simulink model "Potoo_Dyn_Model_v3px4_Flap_compact"  (R2024b)
settings: Solver=FixedStepAuto  StartTime=0.0  StopTime=120  FixedStep=0.001  MaxStep=0.001  RelTol=1e-3
InitFcn:
  | Tmech = 0.004;
undefined symbols (not defined in the file): Control, custom_ff, DiscIntNeverNeededParam, Earth, F, fractalcoef, Light, MIL, Potoo, Px4_Parms, realflap, tau, theta_max, thetadot_max, WGS84
libraries: cstblocks x10, matrix_library x10, aerolibasang x7, simulink x6, aerolibadyn x3, sharedtransform x2, slctrl_autotuning x1, mspfiltlib x1, mspsensorlib x1, shared6dof x1, aerolibactuator x1, aerolibatmos2 x1
(part 2 of 2)

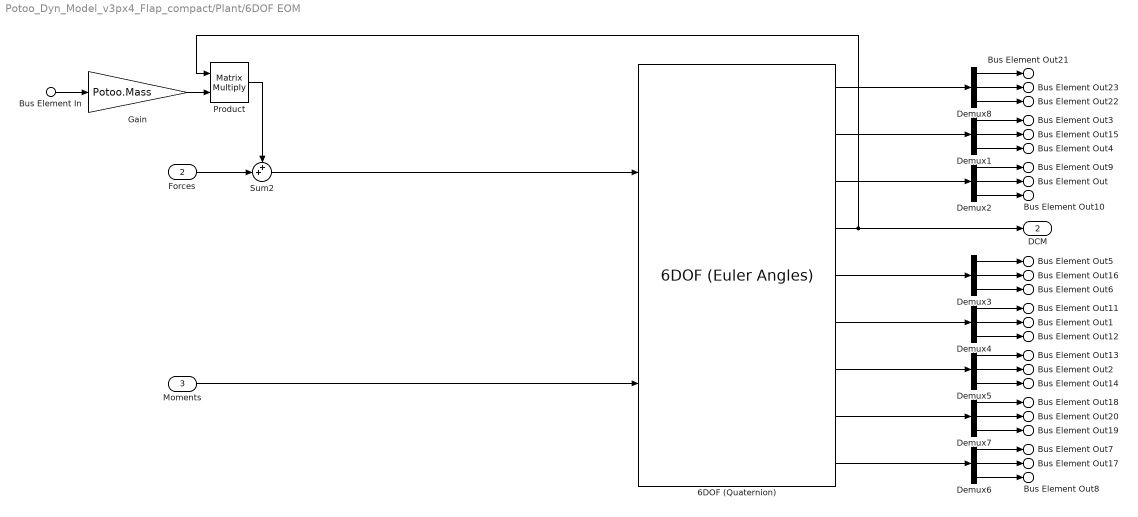
== system Potoo_Dyn_Model_v3px4_Flap_compact/Plant/6DOF EOM ==
  Bus Element In : Inport  PortName=Env  Element=g
  Forces : Inport  Port=2
  Moments : Inport  Port=3
  6DOF (Quaternion) : shared6dof/6DOF (Euler Angles)  units=English (Velocity in ft/s)  mtype=Fixed  rep=Quaternion  xme_0=IC.P_0  Vm_0=IC.V_0  eul_0=IC.E_0  pm_0=IC.omega_0  mass_0=Potoo.Mass  mass_e=0.5  mass_f=2.0  inertia=Potoo.Inertia  inertia_e=eye(3)  inertia_f=2*eye(3)  k_quat=1.0  vre_flag=on  abi_flag=on  aMode=0  xme_statename=''  Vm_statename=''  eul_statename=''  quat_statename=''  pm_statename=''  mass_statename=''
      settings: LibrarySourceBlock=aerolib6dof2/6DOF (Quaternion)
  Demux{1..8} (8 alike) : Demux  Outputs=3
  Gain : Gain  Gain=Potoo.Mass
  Product : Product  Multiplication=Matrix(*)
  Sum2 : Sum  Inputs=++|  InputSameDT=on  SaturateOnIntegerOverflow=on  OutDataTypeStr=Inherit: Same as first input
  Bus Element Out3 : Outport  VectorParamsAs1DForOutWhenUnconnected=off  PortName=States  Element=Xe
  Bus Element Out4 : Outport  VectorParamsAs1DForOutWhenUnconnected=off  PortName=States  Element=Ze
  Bus Element Out : Outport  VectorParamsAs1DForOutWhenUnconnected=off  PortName=States  Element=theta
  Bus Element Out5 : Outport  VectorParamsAs1DForOutWhenUnconnected=off  PortName=States  Element=u
  Bus Element Out6 : Outport  VectorParamsAs1DForOutWhenUnconnected=off  PortName=States  Element=w
  Bus Element Out1 : Outport  VectorParamsAs1DForOutWhenUnconnected=off  PortName=States  Element=q
  Bus Element Out2 : Outport  VectorParamsAs1DForOutWhenUnconnected=off  PortName=States  Element=q_dot
  Bus Element Out7 : Outport  VectorParamsAs1DForOutWhenUnconnected=off  PortName=States  Element=Axe
  Bus Element Out8 : Outport  VectorParamsAs1DForOutWhenUnconnected=off  PortName=States  Element=Aze
  Bus Element Out15 : Outport  VectorParamsAs1DForOutWhenUnconnected=off  PortName=States  Element=Ye
  Bus Element Out9 : Outport  VectorParamsAs1DForOutWhenUnconnected=off  PortName=States  Element=phi
  Bus Element Out10 : Outport  VectorParamsAs1DForOutWhenUnconnected=off  PortName=States  Element=psi
  Bus Element Out16 : Outport  VectorParamsAs1DForOutWhenUnconnected=off  PortName=States  Element=v
  Bus Element Out11 : Outport  VectorParamsAs1DForOutWhenUnconnected=off  PortName=States  Element=p
  Bus Element Out12 : Outport  VectorParamsAs1DForOutWhenUnconnected=off  PortName=States  Element=r
  Bus Element Out13 : Outport  VectorParamsAs1DForOutWhenUnconnected=off  PortName=States  Element=p_dot
  Bus Element Out14 : Outport  VectorParamsAs1DForOutWhenUnconnected=off  PortName=States  Element=r_dot
  Bus Element Out17 : Outport  VectorParamsAs1DForOutWhenUnconnected=off  PortName=States  Element=Aye
  Bus Element Out18 : Outport  VectorParamsAs1DForOutWhenUnconnected=off  PortName=States  Element=u_dot
  Bus Element Out19 : Outport  VectorParamsAs1DForOutWhenUnconnected=off  PortName=States  Element=w_dot
  Bus Element Out20 : Outport  VectorParamsAs1DForOutWhenUnconnected=off  PortName=States  Element=v_dot
  Bus Element Out21 : Outport  VectorParamsAs1DForOutWhenUnconnected=off  PortName=States  Element=Vxe
  Bus Element Out22 : Outport  VectorParamsAs1DForOutWhenUnconnected=off  PortName=States  Element=Vze
  Bus Element Out23 : Outport  VectorParamsAs1DForOutWhenUnconnected=off  PortName=States  Element=Vye
  DCM : Outport  Port=2
  wires:
  Demux6/2 -> Bus Element Out17/1
  Demux6/3 -> Bus Element Out8/1
  Demux6/1 -> Bus Element Out7/1
  Demux5/3 -> Bus Element Out14/1
  Demux5/2 -> Bus Element Out2/1
  Demux5/1 -> Bus Element Out13/1
  Demux4/3 -> Bus Element Out12/1
  Demux4/2 -> Bus Element Out1/1
  Demux4/1 -> Bus Element Out11/1
  Demux3/3 -> Bus Element Out6/1
  Demux3/2 -> Bus Element Out16/1
  Demux3/1 -> Bus Element Out5/1
  Demux2/3 -> Bus Element Out10/1
  Demux2/2 -> Bus Element Out/1
  Demux2/1 -> Bus Element Out9/1
  Demux1/1 -> Bus Element Out3/1
  Demux1/3 -> Bus Element Out4/1
  Demux1/2 -> Bus Element Out15/1
  Forces/1 -> Sum2/2
  Product/1 -> Sum2/1
  6DOF (Quaternion)/8 -> Demux7/1
  6DOF (Quaternion)/9 -> Demux6/1
  6DOF (Quaternion)/2 -> Demux1/1
  6DOF (Quaternion)/3 -> Demux2/1
  6DOF (Quaternion)/7 -> Demux5/1
  6DOF (Quaternion)/6 -> Demux4/1
  6DOF (Quaternion)/5 -> Demux3/1
  Sum2/1 -> 6DOF (Quaternion)/1
  Moments/1 -> 6DOF (Quaternion)/2
  Demux7/3 -> Bus Element Out19/1
  Demux7/2 -> Bus Element Out20/1
  Demux7/1 -> Bus Element Out18/1
  Demux8/1 -> Bus Element Out21/1
  Demux8/3 -> Bus Element Out22/1
  Demux8/2 -> Bus Element Out23/1
  6DOF (Quaternion)/1 -> Demux8/1
  Bus Element In/1 -> Gain/1
  6DOF (Quaternion)/4 -> DCM/1, Product/1
  Gain/1 -> Product/2

== system Potoo_Dyn_Model_v3px4_Flap_compact/Plant/Aerodynamic Model ==
  Env : Inport
  ActuatorCmds : Inport  Port=2  OutDataTypeStr=Bus: ActuatorCmds  PortDimensions=4
  States : Inport  Port=3
  Add : Sum  Inputs=+++++
  Add1 : Sum  Inputs=+++++
  Demux : Demux
  Demux1 : Demux
  For Each Subsystem : Subsystem  TreatAsAtomicUnit=on  mask{wingStruct=[Potoo.Wings.Wing1,Potoo.Wings.Wing2,Potoo.Wings.Wing3,Potoo.Wings.Wing4]}
      mask prompts: wingStruct "Wing Structure"
  Fueslage : Subsystem
  F : Outport  Unit=lbf  VectorParamsAs1DForOutWhenUnconnected=off
  M : Outport  Port=2  Unit=ft*lbf  VectorParamsAs1DForOutWhenUnconnected=off
  wires:
  Add/1 -> F/1
  Add1/1 -> M/1
  States/1 -> For Each Subsystem/3(States)
  ActuatorCmds/1 -> For Each Subsystem/2(Actuator Comands)
  Env/1 -> For Each Subsystem/1(Env)
  For Each Subsystem/1(F) -> Demux/1
  For Each Subsystem/2(M) -> Demux1/1
  Demux/1 -> Add/2
  Demux/2 -> Add/3
  Demux/3 -> Add/4
  Demux/4 -> Add/5
  Demux1/1 -> Add1/1
  Demux1/2 -> Add1/2
  Demux1/3 -> Add1/3
  Demux1/4 -> Add1/4

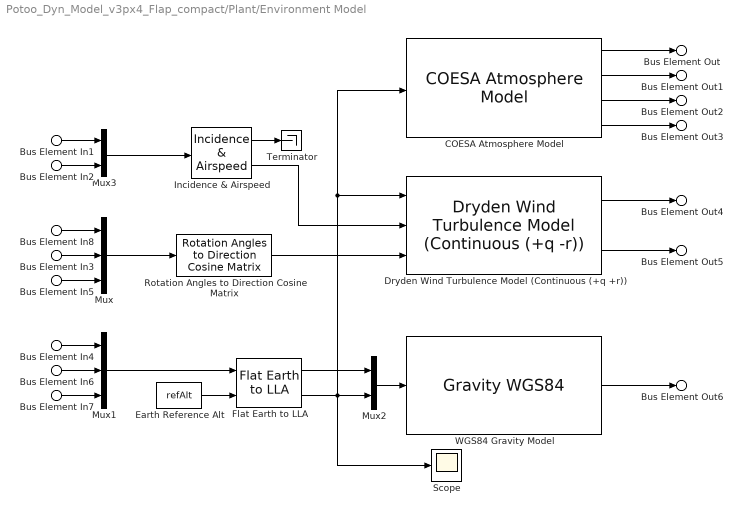
== system Potoo_Dyn_Model_v3px4_Flap_compact/Plant/Environment Model ==
  Bus Element In1 : Inport  PortName=States  Element=u
  Bus Element In2 : Inport  PortName=States  Element=w
  Bus Element In3 : Inport  PortName=States  Element=theta
  Bus Element In4 : Inport  PortName=States  Element=Xe
  Bus Element In7 : Inport  PortName=States  Element=Ze
  Bus Element In8 : Inport  PortName=States  Element=phi
  Bus Element In5 : Inport  PortName=States  Element=psi
  Bus Element In6 : Inport  PortName=States  Element=Ye
  COESA Atmosphere Model : aerolibatmos2/COESA Atmosphere Model  units=English (Velocity in ft/s)  spec=1976 COESA-extended U.S. Standard Atmosphere  model=Profile  profile_var=High temperature  profile_percent=1%  profile_alt=5 km (16404 ft)  envelope_var=High temperature  envelope_percent=1%  action=Warning
  Dryden Wind Turbulence Model (Continuous (+q +r)) : aerolibwind2/Dryden Wind Turbulence Model  (Continuous (+q -r))  units=English (Velocity in ft/s)  spec=MIL-F-8785C  model=Continuous Dryden (+q -r)  W20=W20  Wdeg=Wdeg  TurbProb=10^-2 - Light  L_high=L_high  Wingspan=Wingspan  ts=ts  Seed=Seed  T_on=off
  Earth Reference Alt : Constant  Value=refAlt
  Flat Earth to LLA : aerolibtransform2/Flat Earth to LLA  units=English  ptype=Earth (WGS84)  F=1/298.257223563  R=20925646.3255  refPosPort=off  LL0=[0 0]  psi=0
  Incidence & Airspeed : aerolibasang/Incidence  & Airspeed
  Mux : Mux  Inputs=3
  Mux1 : Mux  Inputs=3
  Mux2 : Mux  Inputs=2
  Mux3 : Mux  Inputs=2
  Rotation Angles to Direction Cosine Matrix : sharedtransform/Rotation Angles to Direction Cosine Matrix  rotationOrder=ZYX  aMode=aMode
  Scope : Scope
  Terminator : Terminator
  "WGS84 Gravity Model  " : GravityWGS84  units=English
  Bus Element Out : Outport  VectorParamsAs1DForOutWhenUnconnected=off  PortName=Env  Element=To
  Bus Element Out1 : Outport  VectorParamsAs1DForOutWhenUnconnected=off  PortName=Env  Element=a
  Bus Element Out2 : Outport  VectorParamsAs1DForOutWhenUnconnected=off  PortName=Env  Element=Po
  Bus Element Out3 : Outport  VectorParamsAs1DForOutWhenUnconnected=off  PortName=Env  Element=AirDensity
  Bus Element Out4 : Outport  VectorParamsAs1DForOutWhenUnconnected=off  PortName=Env  Element=WindVelocity
  Bus Element Out5 : Outport  VectorParamsAs1DForOutWhenUnconnected=off  PortName=Env  Element=WindAngularRates
  Bus Element Out6 : Outport  VectorParamsAs1DForOutWhenUnconnected=off  PortName=Env  Element=g
  wires:
  Dryden Wind Turbulence Model (Continuous (+q +r))/1 -> Bus Element Out4/1
  Dryden Wind Turbulence Model (Continuous (+q +r))/2 -> Bus Element Out5/1
  Mux2/1 -> "WGS84 Gravity Model  "/1
  Bus Element In4/1 -> Mux1/1
  Bus Element In7/1 -> Mux1/3
  Bus Element In6/1 -> Mux1/2
  Bus Element In5/1 -> Mux/3
  Bus Element In8/1 -> Mux/1
  Bus Element In2/1 -> Mux3/2
  Bus Element In1/1 -> Mux3/1
  "WGS84 Gravity Model  "/1 -> Bus Element Out6/1
  COESA Atmosphere Model/2 -> Bus Element Out1/1
  COESA Atmosphere Model/1 -> Bus Element Out/1
  COESA Atmosphere Model/4 -> Bus Element Out3/1
  COESA Atmosphere Model/3 -> Bus Element Out2/1
  Flat Earth to LLA/1 -> Mux2/1
  Earth Reference Alt/1 -> Flat Earth to LLA/2
  Incidence & Airspeed/2 -> Dryden Wind Turbulence Model (Continuous (+q +r))/2
  Flat Earth to LLA/2 -> Scope/1, Mux2/2, COESA Atmosphere Model/1, Dryden Wind Turbulence Model (Continuous (+q +r))/1
  Mux3/1 -> Incidence & Airspeed/1
  Incidence & Airspeed/1 -> Terminator/1
  Mux/1 -> Rotation Angles to Direction Cosine Matrix/1
  Bus Element In3/1 -> Mux/2
  Rotation Angles to Direction Cosine Matrix/1 -> Dryden Wind Turbulence Model (Continuous (+q +r))/3
  Mux1/1 -> Flat Earth to LLA/1

== system Potoo_Dyn_Model_v3px4_Flap_compact/Controller/Attitude Controller/Norm3 ==
  In1 : Inport
  Dot Product : DotProduct  OutDataTypeStr=Inherit: Inherit via internal rule
  Math Function1 : Math  Operator=sqrt  SignedPower=on
  Out1 : Outport  VectorParamsAs1DForOutWhenUnconnected=off
  wires:
  Dot Product/1 -> Math Function1/1
  Math Function1/1 -> Out1/1
  In1/1 -> Dot Product/1, Dot Product/2

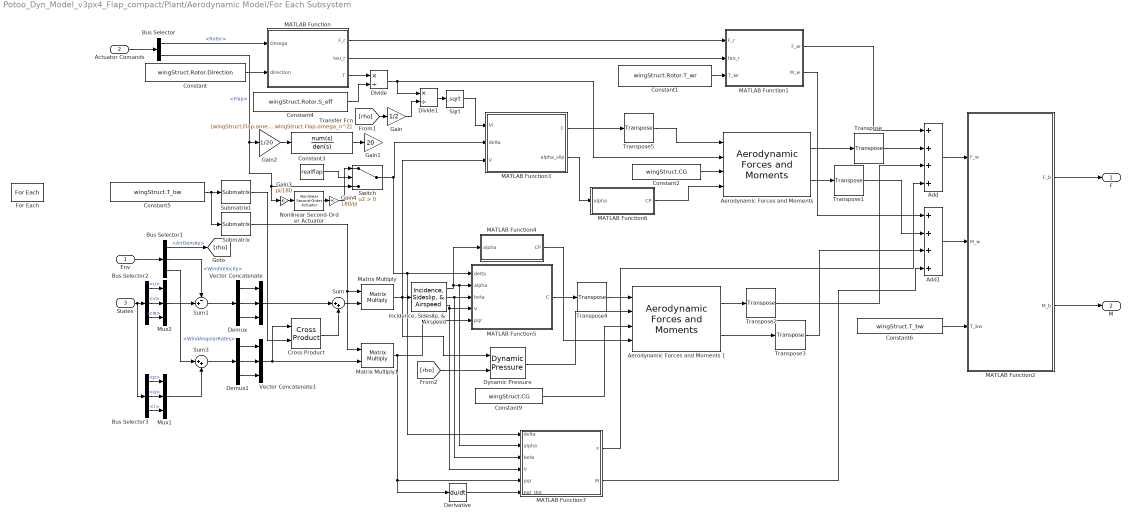
== system Potoo_Dyn_Model_v3px4_Flap_compact/Plant/Aerodynamic Model/For Each Subsystem ==
  Env : Inport
  Actuator Comands : Inport  Port=2  Partition=on  PartitionDimension=1  PartitionWidth=1  PartitionOffset=0
  States : Inport  Port=3
  Add : Sum  Inputs=++++
  Add1 : Sum  Inputs=++++
  "Aerodynamic Forces and Moments " : aerolibadyn/Aerodynamic Forces and Moments   inputAxes=Body  outputForceAxes=Body  outputMomentAxes=Body  S=wingStruct.Rotor.S_eff  b=Potoo.ReferenceSpan  cbar=Potoo.ReferenceLength
  Aerodynamic Forces and Moments 1 : aerolibadyn/Aerodynamic Forces and Moments   inputAxes=Body  outputForceAxes=Body  outputMomentAxes=Body  S=Potoo.ReferenceArea  b=Potoo.ReferenceSpan  cbar=Potoo.ReferenceLength
  Bus Selector : BusSelector  OutputSignals=Rotor,Flap
  Bus Selector1 : BusSelector  OutputSignals=AirDensity,WindVelocity,WindAngularRates
  Bus Selector2 : BusSelector  OutputSignals=u,v,w
  Bus Selector3 : BusSelector  OutputSignals=p,q,r
  Constant : Constant  Value=wingStruct.Rotor.Direction
  Constant1 : Constant  Value=wingStruct.Rotor.T_wr
  Constant2 : Constant  Value=wingStruct.CG
  Constant3 : Constant  Value=realflap
  Constant4 : Constant  Value=wingStruct.Rotor.S_eff
  Constant5 : Constant  Value=wingStruct.T_bw
  Constant6 : Constant  Value=wingStruct.T_bw
  Constant9 : Constant  Value=wingStruct.CG
  Cross Product : matrix_library/Cross Product
  Demux : Demux  Outputs=3
  Demux1 : Demux  Outputs=3
  Derivative : Derivative
  Divide : Product  Inputs=*/
  Divide1 : Product  Inputs=*/
  Dynamic Pressure : aerolibasang/Dynamic Pressure
  For Each : ForEach  DisableCoverage=on  IterateSubsysMaskParameter=on  SubsysMaskParameterIterationDimension=2
  Gain : Gain  Gain=1/2
  Gain1 : Gain  Gain=20
  Gain2 : Gain  Gain=1/20
  Gain3 : Gain  Gain=pi/180
  Gain4 : Gain  Gain=180/pi
  "Incidence, Sideslip, & Airspeed" : aerolibasang/Incidence, Sideslip, & Airspeed
  MATLAB Function : MATLAB Function  TreatAsAtomicUnit=on
  MATLAB Function1 : MATLAB Function  TreatAsAtomicUnit=on
  MATLAB Function2 : MATLAB Function  TreatAsAtomicUnit=on
  MATLAB Function3 : MATLAB Function  TreatAsAtomicUnit=on
  MATLAB Function4 : MATLAB Function  TreatAsAtomicUnit=on
  MATLAB Function5 : MATLAB Function  TreatAsAtomicUnit=on
  MATLAB Function6 : MATLAB Function  TreatAsAtomicUnit=on
  MATLAB Function7 : MATLAB Function  TreatAsAtomicUnit=on
  Matrix Multiply : Product  Multiplication=Matrix(*)
  Matrix Multiply1 : Product  Multiplication=Matrix(*)
  Mux1 : Mux  Inputs=3
  Mux2 : Mux  Inputs=3
  Nonlinear Second-Order Actuator : aerolibactuator/Nonlinear Second-Order Actuator  wn_fin=omega_n  z_fin=zeta  fin_max=theta_max*pi/180  fin_min=-theta_max*pi/180  fin_maxrate=thetadot_max*pi/180  fin_act_0=0  fin_act_vel=0
  Sqrt : Sqrt
  Submatrix : matrix_library/Submatrix  RowSpan=Range of rows  RowStartMode=First  RowStartIndex=1  RowEndMode=Offset from last  RowEndIndex=1  ColSpan=Range of columns  ColStartMode=First  ColStartIndex=1  ColEndMode=Offset from last  ColEndIndex=1
  Submatrix1 : matrix_library/Submatrix  RowSpan=Range of rows  RowStartMode=First  RowStartIndex=1  RowEndMode=Offset from last  RowEndIndex=1  ColSpan=Range of columns  ColStartMode=Last  ColStartIndex=1  ColEndMode=Offset from last  ColEndIndex=1
  Sum : Sum  Inputs=|++
  Sum1 : Sum  Inputs=-+|  InputSameDT=on  SaturateOnIntegerOverflow=on  OutDataTypeStr=Inherit: Same as first input
  Sum3 : Sum  Inputs=|++  InputSameDT=on  SaturateOnIntegerOverflow=on  OutDataTypeStr=Inherit: Same as first input
  Switch : Switch  Criteria=u2 > Threshold  SaturateOnIntegerOverflow=off  InputSameDT=off
  Transfer Fcn : TransferFcn  Numerator=[wingStruct.Flap.omega_n^2]  Denominator=[1 2*wingStruct.Flap.omega_n wingStruct.Flap.omega_n^2]
  Transpose{,1..5} (6 alike) : matrix_library/Transpose
  Vector Concatenate : Concatenate  NumInputs=3
  Vector Concatenate1 : Concatenate  NumInputs=3
  F : Outport  Unit=N  ConcatenationDimension=1  VectorParamsAs1DForOutWhenUnconnected=off
  M : Outport  Port=2  Unit=N*m  ConcatenationDimension=1  VectorParamsAs1DForOutWhenUnconnected=off
  wires:
  Bus Selector3/2 -> Mux1/2  "<q>"
  Bus Selector2/2 -> Mux2/2  "<v>"
  Bus Selector3/3 -> Mux1/3  "<r>"
  Bus Selector1/3 -> Sum3/1  "<WindAngularRates>"
  Bus Selector2/1 -> Mux2/1  "<u>"
  Env/1 -> Bus Selector1/1
  [rho] -> Dynamic Pressure/2
  Bus Selector2/3 -> Mux2/3  "<w>"
  States/1 -> Bus Selector3/1, Bus Selector2/1
  Bus Selector1/1 -> [rho]  "<AirDensity>"
  MATLAB Function/2(tau_r) -> MATLAB Function1/2(tau_r)
  MATLAB Function2/2(M_b) -> M/1
  Mux2/1 -> Sum1/2
  Constant2/1 -> "Aerodynamic Forces and Moments "/3
  Demux1/1 -> Vector Concatenate1/1
  Transpose3/1 -> Add1/3
  Constant4/1 -> Divide/2
  Dynamic Pressure/1 -> Aerodynamic Forces and Moments 1/2
  Demux/2 -> Vector Concatenate/2
  "Aerodynamic Forces and Moments "/2 -> Transpose1/1
  Sum3/1 -> Demux1/1
  Demux/3 -> Vector Concatenate/3
  Constant6/1 -> MATLAB Function2/3(T_bw)
  Sum1/1 -> Demux/1
  "Incidence, Sideslip, & Airspeed"/2 -> MATLAB Function5/3(beta), MATLAB Function7/3(beta)
  Add1/1 -> MATLAB Function2/2(M_w)
  Mux1/1 -> Sum3/2
  Demux1/3 -> Vector Concatenate1/3
  MATLAB Function5/1(C) -> Transpose4/1
  MATLAB Function1/2(M_w) -> Add1/1
  Submatrix/1 -> Matrix Multiply/1, Matrix Multiply1/1
  MATLAB Function1/1(F_w) -> Add/1
  Transpose4/1 -> Aerodynamic Forces and Moments 1/1
  MATLAB Function3/1(C) -> Transpose5/1
  Add/1 -> MATLAB Function2/1(F_w)
  Transpose1/1 -> Add1/2
  Constant/1 -> MATLAB Function/2(direction)
  Matrix Multiply1/1 -> MATLAB Function7/5(pqr), Derivative/1, MATLAB Function5/5(pqr)
  Actuator Comands/1 -> Bus Selector/1
  MATLAB Function/3(T) -> Divide/1
  Sum/1 -> Matrix Multiply/2
  Vector Concatenate1/1 -> Matrix Multiply1/2, Cross Product/1
  Demux/1 -> Vector Concatenate/1
  Constant5/1 -> Submatrix/1, Submatrix1/1
  Constant1/1 -> MATLAB Function1/3(T_wr)
  Transpose/1 -> Add/2
  "Incidence, Sideslip, & Airspeed"/3 -> MATLAB Function5/4(V), MATLAB Function7/4(V)
  Divide/1 -> Divide1/1, "Aerodynamic Forces and Moments "/2
  "Aerodynamic Forces and Moments "/1 -> Transpose/1
  Submatrix1/1 -> Cross Product/2
  Matrix Multiply/1 -> MATLAB Function3/3(V), "Incidence, Sideslip, & Airspeed"/1, Dynamic Pressure/1
  Constant9/1 -> Aerodynamic Forces and Moments 1/3
  MATLAB Function2/1(F_b) -> F/1
  Bus Selector3/1 -> Mux1/1  "<p>"
  Cross Product/1 -> Sum/2
  Demux1/2 -> Vector Concatenate1/2
  MATLAB Function4/1(CP) -> Aerodynamic Forces and Moments 1/4
  Vector Concatenate/1 -> Sum/1
  Aerodynamic Forces and Moments 1/1 -> Transpose2/1
  MATLAB Function/1(F_r) -> MATLAB Function1/1(F_r)
  Bus Selector1/2 -> Sum1/1  "<WindVelocity>"
  Aerodynamic Forces and Moments 1/2 -> Transpose3/1
  Bus Selector/1 -> MATLAB Function/1(Omega)  "<Rotor>"
  Transpose2/1 -> Add/3
  Transpose5/1 -> "Aerodynamic Forces and Moments "/1
  [rho] -> Gain/1
  Gain/1 -> Divide1/2
  Divide1/1 -> Sqrt/1
  Sqrt/1 -> MATLAB Function3/1(Vi)
  MATLAB Function6/1(CP) -> "Aerodynamic Forces and Moments "/4
  "Incidence, Sideslip, & Airspeed"/1 -> MATLAB Function5/2(alpha), MATLAB Function7/2(alpha), MATLAB Function4/1(alpha)
  MATLAB Function3/2(alpha_slip) -> MATLAB Function6/1(alpha)
  Bus Selector/2 -> Gain2/1, Switch/3, Gain3/1  "<Flap>"
  MATLAB Function7/1(F) -> Add/4
  MATLAB Function7/2(M) -> Add1/4
  Derivative/1 -> MATLAB Function7/6(pqr_dot)
  Gain2/1 -> Transfer Fcn/1
  Transfer Fcn/1 -> Gain1/1
  Switch/1 -> MATLAB Function7/1(delta), MATLAB Function5/1(delta), MATLAB Function3/2(delta)
  Constant3/1 -> Switch/2
  Gain3/1 -> Nonlinear Second-Order Actuator/1
  Nonlinear Second-Order Actuator/1 -> Gain4/1
  Gain4/1 -> Switch/1

== system Potoo_Dyn_Model_v3px4_Flap_compact/Plant/Aerodynamic Model/Fueslage ==
  Bus Element In14 : Inport  PortName=Env  Element=WindVelocity
  Bus Element In15 : Inport  PortName=Env  Element=WindAngularRates
  Bus Element In7 : Inport  PortName=Env  Element=AirDensity
  Bus Element In1 : Inport  Port=2  PortName=States  Element=u
  Bus Element In2 : Inport  Port=2  PortName=States  Element=w
  Bus Element In3 : Inport  Port=2  PortName=States  Element=q
  Bus Element In6 : Inport  Port=2  PortName=States  Element=v
  Bus Element In4 : Inport  Port=2  PortName=States  Element=p
  Bus Element In5 : Inport  Port=2  PortName=States  Element=r
  "Aerodynamic Forces and Moments " : aerolibadyn/Aerodynamic Forces and Moments   inputAxes=Body  outputForceAxes=Body  outputMomentAxes=Body  S=pi/4*(8/12)^2  b=8/12  cbar=20/12
  Constant : Constant  Value=[0,0,0]
  Demux : Demux  Outputs=3
  Demux1 : Demux  Outputs=3
  Dynamic Pressure : aerolibasang/Dynamic Pressure
  "Incidence, Sideslip, & Airspeed" : aerolibasang/Incidence, Sideslip, & Airspeed
  MATLAB Function5 : MATLAB Function  TreatAsAtomicUnit=on
  Mux1 : Mux  Inputs=3
  Mux2 : Mux  Inputs=3
  Sum1 : Sum  Inputs=-+|  InputSameDT=on  SaturateOnIntegerOverflow=on  OutDataTypeStr=Inherit: Same as first input
  Sum3 : Sum  Inputs=|++  InputSameDT=on  SaturateOnIntegerOverflow=on  OutDataTypeStr=Inherit: Same as first input
  Transpose : matrix_library/Transpose
  Vector Concatenate : Concatenate  NumInputs=3
  Vector Concatenate1 : Concatenate  NumInputs=3
  F : Outport  Unit=N  VectorParamsAs1DForOutWhenUnconnected=off
  M : Outport  Port=2  Unit=N*m  VectorParamsAs1DForOutWhenUnconnected=off
  wires:
  Sum3/1 -> Demux1/1
  Demux1/1 -> Vector Concatenate1/1
  Demux1/2 -> Vector Concatenate1/2
  Demux1/3 -> Vector Concatenate1/3
  Demux/3 -> Vector Concatenate/3
  Demux/2 -> Vector Concatenate/2
  Demux/1 -> Vector Concatenate/1
  Sum1/1 -> Demux/1
  Bus Element In2/1 -> Mux2/3
  Bus Element In15/1 -> Sum3/1
  Mux1/1 -> Sum3/2
  Bus Element In3/1 -> Mux1/2
  Bus Element In4/1 -> Mux1/1
  Bus Element In6/1 -> Mux2/2
  Bus Element In1/1 -> Mux2/1
  Bus Element In5/1 -> Mux1/3
  Mux2/1 -> Sum1/2
  Bus Element In14/1 -> Sum1/1
  Vector Concatenate/1 -> Dynamic Pressure/1, "Incidence, Sideslip, & Airspeed"/1
  "Incidence, Sideslip, & Airspeed"/1 -> MATLAB Function5/1(alpha)
  "Incidence, Sideslip, & Airspeed"/2 -> MATLAB Function5/2(beta)
  Vector Concatenate1/1 -> MATLAB Function5/3(pqr)
  Bus Element In7/1 -> Dynamic Pressure/2
  MATLAB Function5/1(C) -> Transpose/1
  Dynamic Pressure/1 -> "Aerodynamic Forces and Moments "/2
  Constant/1 -> "Aerodynamic Forces and Moments "/3, "Aerodynamic Forces and Moments "/4
  "Aerodynamic Forces and Moments "/2 -> M/1
  "Aerodynamic Forces and Moments "/1 -> F/1
  Transpose/1 -> "Aerodynamic Forces and Moments "/1

== matlab function Potoo_Dyn_Model_v3px4_Flap_compact/Controller/MATLAB Function2 ==
  settings: updateMethod=DISCRETE
  data: F1 input; F1 output; F2 input; F3 input; F4 input; F2 output; F3 output; F4 output; t input; mission input
function [F1,F2,F3,F4] = Mission_Cmd(F1,F2,F3,F4,t,mission)

persistent t_flag state i j
if isempty(t_flag)
    t_flag = t;
    state = 0;
    i = 1;
    j = 1;
end

% mission = 0;

if mission == 1
    recover = 5;
    actuate = 8;
    
    delta_max = 10;
    
    switch state
        case 0
            if t >= t_flag+recover
                t_flag = t;
                state = 1;
            end
        case 1
            if t >= t_flag+actuate
                t_flag = t;
                state = 0;
                j = j*-1;
                if j == 1
                    i = i+1;
                end
            end
            if i <= 4
                F1 = j*i*0.25*delta_max;
                F2 = j*i*0.25*delta_max;
                F3 = 0;
                F4 = 0;
            end
    end

elseif mission == 2
    delta_max = 20;
    tau = 0.5; % sec
    % t_0 = 15; % sec
    recover = 10;

    % if t >= t_0 && t <= t_0+tau
    %     F3 = delta_max*sin(2*pi/tau*(t-t_0));
    %     F4 = -delta_max*sin(2*pi/tau*(t-t_0));
    %     F1 = 0;
    %     F2 = 0;
    % else
    % 
    % end
    switch state
        case 0
            if t >= t_flag+recover
                t_flag = t;
                state = 1;
            end
        case 1
            if t >= t_flag+tau
                t_flag = t;
                state = 0;
                j = j*-1;
                if j == 1
                    i = i+1;
                end
            end
            if i <= 4
                F3 = j*i*0.25*delta_max*sin(2*pi/tau*(t-t_flag));
                F4 = j*i*0.25*delta_max*-sin(2*pi/tau*(t-t_flag));
                F1 = 0;
                F2 = 0;
            end
    end

% elseif mission == 0
%     if t>=5 && t<6
%         F3 = 20;
%         F4 = -20;
%         F1 = 0;
%         F2 = 0;
%     end

else

end

end

== matlab function Potoo_Dyn_Model_v3px4_Flap_compact/Plant/Aerodynamic Model/Fueslage/MATLAB Function5 ==
  data: C output; alpha input; beta input; pqr input
function C  = Aero_Coef_V2(alpha,beta,pqr)

% State Vector
x = [alpha;beta;pqr];

% Aero Constants
c_Lalpha = 0.001*180/pi;
c_Sbeta = 0.001*180/pi;
c_L0 = 0;
c_D0 = 0.01;
c_malpha = 0.0001*180/pi;
c_mbeta = 0.0001*180/pi;
AR = 8/20;
e = 0.25;

% AoA
C_Xalpha = c_Lalpha*alpha+c_L0-(2/(pi*AR*e)*(c_Lalpha*alpha+c_L0).*c_Lalpha);
C_Yalpha = 0;
C_Zalpha = -c_Lalpha-(1/(pi*AR*e)*(c_Lalpha*alpha+c_L0).^2+c_D0);
C_lalpha = 0;
C_malpha = c_malpha;
C_nalpha = 0;
C_alpha = [C_Xalpha,C_Yalpha,C_Zalpha,C_lalpha,C_malpha,C_nalpha]';

% Sideslip
C_Xbeta = c_Sbeta*beta-(2/(pi*AR*e)*(c_Sbeta*beta).*c_Sbeta);
C_Ybeta = -c_Sbeta-(1/(pi*AR*e)*(c_Sbeta*beta).^2+c_D0);
C_Zbeta = 0;
C_lbeta = 0;
C_mbeta = c_mbeta;
C_nbeta = 0;
C_beta = [C_Xbeta,C_Ybeta,C_Zbeta,C_lbeta,C_mbeta,C_nbeta]';

% Roll Rate
C_Xp = 0;
C_Yp = 0;
C_Zp = 0;
C_lp = 0;
C_mp = 0;
c_np = 0;
C_p = [C_Xp,C_Yp,C_Zp,50*C_lp,C_mp,c_np]';

% Pitch Rate
C_Xq = 0;
C_Yq = 0;
C_Zq = 2*0.25*c_Lalpha;
C_lq = 0;
C_mq = -2*0.25^2*c_Lalpha;
C_nq = 0;
C_q = [C_Xq,C_Yq,C_Zq,C_lq,C_mq,C_nq]';

% Yaw Rate
C_Xr = 0;
C_Yr = 0;
C_Zr = 0;
C_lr = 0;
C_mr = 0;
C_nr = 0;
C_r = [C_Xr,C_Yr,C_Zr,C_lr,C_mr,C_nr]';

% Combined
A = [C_alpha,C_beta,C_p,C_q,C_r];
C = A*x;

end

== matlab function Potoo_Dyn_Model_v3px4_Flap_compact/Controller/Subsystem/Integrate Angular Velocity ==
  data: av input; q output; rate parameter
function q = integrateAngVel(av, rate)
%INTEGRATEANGVEL Integrate angular velocity to a quaternion
%  Treat Angular Velocity as an incremental rotation vector.

%   Copyright 2019 The MathWorks, Inc.   

persistent orient
if isempty(orient)
    % Initial orientation is the identity quaternion.
    orient = cast(quaternion(1,0,0,0), 'like', av);
end

% Convert angular velocity to a rotation vector.
rv = quaternion(av*(1/rate), 'rotvec');
orient = rv * orient;
q = compact(orient);

== matlab function Potoo_Dyn_Model_v3px4_Flap_compact/Plant/Aerodynamic Model/For Each Subsystem/MATLAB Function ==
  data: Omega input; F_r output; tau_r output; direction input; T output
function [F_r,tau_r,T] = Rotor_Loads(Omega,direction)

k = direction;

k_T.P2 = 1.264*10^-7;   % lbf/RPM^2 

k_tau.P2 = 7.766*10^-9;     % (ft-lbf)/RPM^2

T = k_T.P2*Omega^2;
tau = -k*(k_tau.P2*Omega^2);

% F_r = [0,0,T]';
% tau_r = [0,0,tau]';
F_r = [T,0,0]';
tau_r = [tau,0,0]';

end

== matlab function Potoo_Dyn_Model_v3px4_Flap_compact/Plant/Aerodynamic Model/For Each Subsystem/MATLAB Function1 ==
  data: F_r input; F_w output; M_w output; tau_r input; T_wr input
function [F_w,M_w] = WingAxis_Loads(F_r,tau_r,T_wr)

R = T_wr(1:3,1:3);
R = R';
P = T_wr(1:3,4);

F_w = R*F_r;
M_w = R*tau_r+cross(P,F_w);

end

== matlab function Potoo_Dyn_Model_v3px4_Flap_compact/Plant/Aerodynamic Model/For Each Subsystem/MATLAB Function2 ==
  data: F_w input; F_b output; M_b output; M_w input; T_bw input
function [F_b,M_b] = BodyAxis_Loads(F_w,M_w,T_bw)

R = T_bw(1:3,1:3);
R = R';
P = T_bw(1:3,4);

F_b = R*F_w;
M_b = R*M_w+cross(P,F_b);

end

== matlab function Potoo_Dyn_Model_v3px4_Flap_compact/Plant/Aerodynamic Model/For Each Subsystem/MATLAB Function3 ==
  data: Vi input; delta input; C output; V input; alpha_slip output
function [C,alpha_slip]  = Hover_Coef(Vi,delta,V)

Vx = V(3);
if Vi == 0
    alpha_slip = 0;
else
    alpha_slip = atan(Vx/Vi);
end

x = [delta,alpha_slip]';

% Geometric Constants
D = 15/12;
c = 15.5/12;
AR = D/c;

% Aero Constants
c_Lalpha = 0.062*180/pi;
c_Lalpha = c_Lalpha*(AR+2)/(AR+3.54);
c_L0 = 0;
c_m0 = 0;
c_malpha = 0.0008*180/pi;
e = 0.7;

% Flap Deflection
C_Xdelta = -0.0002;
C_Ydelta = 0;
C_Zdelta = -0.024;
C_ldelta = 0;
C_mdelta = -0.011;
C_ndelta = 0;
C_delta = [C_Xdelta,C_Ydelta,C_Zdelta,C_ldelta,C_mdelta,C_ndelta]';

% AoA
C_L = c_Lalpha*alpha_slip+c_L0;
C_m = c_malpha*alpha_slip+c_m0;
C_D0 = 0.007+0.95*alpha_slip^2;
C_Di = C_L^2/(pi*AR*e);
C_D = C_D0+C_Di;

if alpha_slip == 0
    C_Xalpha = -C_D;
    C_Yalpha = 0;
    C_Zalpha = -C_L;
    C_lalpha = 0;
    C_malpha = C_m;
    C_nalpha = 0;
    C_alpha = [C_Xalpha,C_Yalpha,C_Zalpha,C_lalpha,C_malpha,C_nalpha]';
else
    C_N = C_L*cos(alpha_slip)+C_D*sin(alpha_slip);
    C_A = C_D*cos(alpha_slip)-C_L*sin(alpha_slip);

    C_Xalpha = -C_A;
    C_Yalpha = 0;
    C_Zalpha = -C_N;
    C_lalpha = 0;
    C_malpha = C_m;
    C_nalpha = 0;
    C_alpha = [C_Xalpha,C_Yalpha,C_Zalpha,C_lalpha,C_malpha,C_nalpha]'/alpha_slip; 
end


A = [C_delta,C_alpha];
C = A*x;

if alpha_slip == 0
    C = C+C_alpha;
end

end

== matlab function Potoo_Dyn_Model_v3px4_Flap_compact/Plant/Aerodynamic Model/For Each Subsystem/MATLAB Function4 ==
  data: alpha input; CP output
function CP = Cp_shift(alpha)

alpha_0 = 0;
c = 15.5/12;

if (abs(alpha)*180/pi-alpha_0) < 20
    X_cp = 0.25*c;
elseif (alpha*180/pi-alpha_0) >= 20 && (alpha*180/pi-alpha_0) <= 160
    X_cp = (0.33+0.0019*(alpha-alpha_0))*c;
elseif (alpha*180/pi-alpha_0) <= -20 && (alpha*180/pi-alpha_0) >= -160
    X_cp = (0.33-0.0019*(alpha-alpha_0))*c;
else
    X_cp = 0.5*c;
end

CP = [X_cp,0,0];

end

== matlab function Potoo_Dyn_Model_v3px4_Flap_compact/Plant/Aerodynamic Model/For Each Subsystem/MATLAB Function5 ==
  data: delta input; C output; alpha input; beta input; V input; pqr input
function C  = Aero_Coef_V4(delta,alpha,beta,V,pqr)

% Geometric Constants
b = 2;
c = 15.5/12;
AR = b/c;

% Aero Constants
c_Lalpha = 0.062*180/pi;
c_L0 = 0;
c_m0 = 0;
c_malpha = 0.0008*180/pi;
e = 0.7;

% State Vector
p = pqr(1);
q = pqr(2);
r = pqr(3);

    if V > 0
        pbar = p*b/(2*V);
        qbar = q*c/(2*V);
        rbar = r*b/(2*V);
    else
        pbar = 0;
        qbar = 0;
        rbar = 0;
    end

x = [delta;alpha;beta;pbar;qbar;rbar];

% Flap Deflection
C_Xdelta = -0.0002;
C_Ydelta = 0;
C_Zdelta = -0.024;
C_ldelta = 0;
C_mdelta = -0.011;
C_ndelta = 0;
C_delta = [C_Xdelta,C_Ydelta,C_Zdelta,C_ldelta,C_mdelta,C_ndelta]';

% AoA
A = 1.1;
B = -0.5;
F = 0.11;
D = 1.135;
E = -1.05;
alpha_0 = 0;
if abs(alpha)*180/pi <= 15
    C_L = c_Lalpha*alpha+c_L0;
    C_m = c_malpha*alpha+c_m0;
    C_D0 = 0.007+0.95*alpha^2;
    C_Di = C_L^2/(pi*AR*e);
    C_D = C_D0+C_Di;

    if alpha == 0
        C_Xalpha = -C_D;
        C_Yalpha = 0;
        C_Zalpha = -C_L;
        C_lalpha = 0;
        C_malpha = C_m;
        C_nalpha = 0;
        C_alpha = [C_Xalpha,C_Yalpha,C_Zalpha,C_lalpha,C_malpha,C_nalpha]';
    else
        C_N = C_L*cos(alpha)+C_D*sin(alpha);
        C_A = C_D*cos(alpha)-C_L*sin(alpha);

        C_Xalpha = -C_A;
        C_Yalpha = 0;
        C_Zalpha = -C_N;
        C_lalpha = 0;
        C_malpha = C_m;
        C_nalpha = 0;
        C_alpha = [C_Xalpha,C_Yalpha,C_Zalpha,C_lalpha,C_malpha,C_nalpha]'/alpha; 
    end
elseif abs(alpha*180/pi) > 15 && abs(alpha*180/pi) <= 20
    C_L20 = A*sin(2*(20*pi/180-alpha_0));
    C_m20 = B*sin(20*pi/180-alpha_0)+F*sin(2*(20*pi/180-alpha_0));
    C_D20 = D + E*cos(2*(30*pi/180-alpha_0));

    C_L15 = c_Lalpha*15*pi/180+c_L0;
    C_m15 = c_malpha*15*pi/180+c_m0;
    C_D0 = 0.007+0.95*(15*pi/180)^2;
    C_Di = C_L15^2/(pi*AR*e);
    C_D15 = C_D0+C_Di;

    k_L = (C_L20-C_L15)/(5*pi/180);
    k_m = (C_m20-C_m15)/(5*pi/180);
    k_D = (C_D20-C_D15)/(5*pi/180);

    C_L = (C_L15+k_L*(abs(alpha)-15*pi/180))*alpha/abs(alpha);
    C_m = (C_m15+k_m*(abs(alpha)-15*pi/180))*alpha/abs(alpha);
    C_D = C_D15+k_D*(abs(alpha)-15*pi/180);

    C_N = C_L*cos(alpha)+C_D*sin(alpha);
    C_A = C_D*cos(alpha)-C_L*sin(alpha);

    C_Xalpha = -C_A;
    C_Yalpha = 0;
    C_Zalpha = -C_N;
    C_lalpha = 0;
    C_malpha = C_m;
    C_nalpha = 0;
    C_alpha = [C_Xalpha,C_Yalpha,C_Zalpha,C_lalpha,C_malpha,C_nalpha]'/alpha; 
else
    C_L = A*sin(2*(alpha-alpha_0));
    C_m = B*sin(alpha-alpha_0)+F*sin(2*(alpha-alpha_0));
    C_D = D + E*cos(2*(alpha-alpha_0));

    C_N = C_L*cos(alpha)+C_D*sin(alpha);
    C_A = C_D*cos(alpha)-C_L*sin(alpha);

    C_Xalpha = -C_A;
    C_Yalpha = 0;
    C_Zalpha = -C_N;
    C_lalpha = 0;
    C_malpha = C_m;
    C_nalpha = 0;
    C_alpha = [C_Xalpha,C_Yalpha,C_Zalpha,C_lalpha,C_malpha,C_nalpha]'/alpha; 
end

% Sideslip
C_Xbeta = 0;
C_Ybeta = 0;
C_Zbeta = 0;
C_lbeta = 0;
C_mbeta = 0;
C_nbeta = 0;
C_beta = [C_Xbeta,C_Ybeta,C_Zbeta,C_lbeta,C_mbeta,C_nbeta]';

% Roll Rate
k_lp = (1+c_Lalpha/(pi*AR))/(1+2*c_Lalpha/(pi*AR));
C_Xp = 0;
C_Yp = 0;
C_Zp = 0;
C_mp = 0;
if V == 0
    C_lp = 0;
    C_np = 0;
else
    C_lp = -k_lp*b/(16*V)*c_Lalpha;
    C_np = -(1-3*k_lp/(pi*AR)*c_Lalpha)*(c_Lalpha*alpha+c_L0)*b/(16*V);
end
C_p = [C_Xp,C_Yp,C_Zp,C_lp,C_mp,C_np]';


% Pitch Rate
C_Xq = 0;
C_Yq = 0;
% C_Zq = 2*0.1*c_Lalpha;
C_Zq = 0;
C_lq = 0;
% C_mq = -2*0.1^2*c_Lalpha;
C_mq = -0;
C_nq = 0;
C_q = [C_Xq,C_Yq,C_Zq,C_lq,C_mq,C_nq]';

% Yaw Rate
C_Xr = 0;
C_Yr = 0;
C_Zr = 0;
C_lr = (1-3*k_lp/(pi*AR)*c_Lalpha)*(c_Lalpha*alpha+c_L0)/4;
C_mr = 0;
C_nr = 0;
C_r = [C_Xr,C_Yr,C_Zr,C_lr,C_mr,C_nr]';

% Combined
A = [C_delta,C_alpha,C_beta,C_p,C_q,C_r];
C = A*x;

if alpha == 0
    C = C+C_alpha;
end

end

== matlab function Potoo_Dyn_Model_v3px4_Flap_compact/Plant/Aerodynamic Model/For Each Subsystem/MATLAB Function6 ==
  data: alpha input; CP output
function CP = Cp_shift(alpha)

alpha_0 = 0;
c = 15.5/12;

if (abs(alpha)*180/pi-alpha_0) < 20
    X_cp = 0.25*c;
elseif (alpha*180/pi-alpha_0) >= 20 && (alpha*180/pi-alpha_0) <= 160
    X_cp = (0.33+0.0019*(alpha-alpha_0))*c;
elseif (alpha*180/pi-alpha_0) <= -20 && (alpha*180/pi-alpha_0) >= -160
    X_cp = (0.33-0.0019*(alpha-alpha_0))*c;
else
    X_cp = 0.5*c;
end

CP = [X_cp,0,0];

end

== matlab function Potoo_Dyn_Model_v3px4_Flap_compact/Controller/MATLAB Function3 ==
  data: delta input; thrust input; R1 output; R2 output; R3 output; R4 output; mix input
function [R1,R2,R3,R4] = RotorControlMixing(delta,thrust,mix)

k_T = 1.264*10^-7;   % lbf/RPM^2 

T = thrust/4;
T = T*0.22; % N to lbf
omega = sqrt(T/k_T);

m = 0.3;
% c_T = .01;
% rho = 1.225;
% r = 15/2*0.0254;
% A = pi*r^2;
% omega = sqrt(T/4/(c_T*rho*A))/r;


Roll = sqrt(abs(delta(1))/m*0.22/k_T)*sign(delta(1));
Pitch = sqrt(abs(delta(2))/m*0.22/k_T)*sign(delta(2));
Yaw = sqrt(abs(delta(3))/m*0.22/k_T)*sign(delta(3));
% Roll = 0;
% Pitch = 0;
% Yaw = 0;
% Collective = omega*180/pi;
Collective = omega;

cmd = [Collective,Roll,Pitch,Yaw]';
cntrl = mix*cmd;

R1 = cntrl(1);
R2 = cntrl(2);
R3 = cntrl(3);
R4 = cntrl(4);


end

== matlab function Potoo_Dyn_Model_v3px4_Flap_compact/Controller/MATLAB Function4 ==
  data: delta input; R1 output; R2 output; R3 output; R4 output; mix input
function [R1,R2,R3,R4] = FlapControlMixing(delta,mix)

m = 20/0.375;

Roll = m*delta(1);
Pitch = m*delta(2);
Yaw = m*delta(3);

cmd = [Roll,Pitch,Yaw]';
cntrl = mix*cmd;

R1 = cntrl(1);
R2 = cntrl(2);
R3 = cntrl(3);
R4 = cntrl(4);

end

== matlab function Potoo_Dyn_Model_v3px4_Flap_compact/Controller/Attitude Controller/MATLAB Function ==
  data: body_z input; q_sp output; yaw_sp input
function q_sp = bodyz2attitude(body_z,yaw_sp)

if dot(body_z,body_z) == 0
    body_z(3) = 1;
end
body_z = body_z/sqrt(dot(body_z,body_z));

y_c = [-sin(yaw_sp),cos(yaw_sp),0]';
body_x = cross(y_c,body_z);
if body_z(3) < 0
    body_x = -body_x;
elseif body_z(3) == 0
    body_x = [0 0 1]';
end
body_x = body_x/sqrt(dot(body_x,body_x));

body_y = cross(body_z,body_x);

R_sp = [body_x,body_y,body_z];

q_sp = rotm2quat(R_sp);

== matlab function Potoo_Dyn_Model_v3px4_Flap_compact/Controller/Angle Controller/MATLAB Function ==
  data: q_sp input; q_e0 output; att input; q_ev output
function [q_e0,q_ev] = quat_error(q_sp,att)

eul = [att(3),att(1),att(2)];
q = eul2quat(eul);

Q = [q(1),-q(2),-q(3),-q(4);...
    q(2),q(1),-q(4),q(3);...
    q(3),q(4),q(1),-q(2);...
    q(4),-q(3),q(2),q(1)];

q_e = Q*q_sp';
q_e0 = q_e(1);
q_ev = q_e(2:end);

== matlab function Potoo_Dyn_Model_v3px4_Flap_compact/Controller/MATLAB Function ==
  data: eul input; quat output
function quat = quat_sp(eul)

phi = eul(1);
theta = eul(2);
psi = eul(3);

eul = [psi,theta,phi];
quat = eul2quat(eul,"ZYX");

== matlab function Potoo_Dyn_Model_v3px4_Flap_compact/Plant/Aerodynamic Model/For Each Subsystem/MATLAB Function7 ==
  data: delta input; F output; alpha input; beta input; V input; pqr input; M output; pqr_dot input
function [F,M]  = Aero_FM_misc(delta,alpha,beta,V,pqr,pqr_dot)

% Geometric Constants
b = 2;
c = 15.5/12;
AR = b/c;

% Aero Constants
c_Lalpha = 0.062*180/pi;
c_L0 = 0;
c_m0 = 0;
c_malpha = 0.0008*180/pi;
e = 0.7;

% State Vector
p = pqr(1);
q = pqr(2);
r = pqr(3);

%     if V > 0
%         pbar = p*b/(2*V);
%         qbar = q*c/(2*V);
%         rbar = r*b/(2*V);
%     else
%         pbar = 0;
%         qbar = 0;
%         rbar = 0;
%     end
% p_dot = pqr_dot(1);
% q_dot = pqr_dot(2);
% r_dot = pqr_dot(3);
%     if V > 0
%         p_dot = p_dot*b/(2*V);
%         q_dot = q_dot*c/(2*V);
%         r_dot = r_dot*b/(2*V);
%     else
%         p_dot = 0;
%         q_dot = 0;
%         r_dot = 0;
%     end

% x = [delta;alpha;beta;pbar;qbar;rbar];
% x = [delta;alpha;beta;pbar;qbar;rbar;p_dot;q_dot;r_dot];
x = [delta;alpha;beta;p;q;r];

% Flap Deflection
C_Xdelta = 0;
C_Ydelta = 0;
C_Zdelta = 0;
C_ldelta = 0;
C_mdelta = 0;
C_ndelta = 0;
C_delta = [C_Xdelta,C_Ydelta,C_Zdelta,C_ldelta,C_mdelta,C_ndelta]';

% AoA
C_Xalpha = 0;
C_Yalpha = 0;
C_Zalpha = 0;
C_lalpha = 0;
C_malpha = 0;
C_nalpha = 0;
C_alpha = [C_Xalpha,C_Yalpha,C_Zalpha,C_lalpha,C_malpha,C_nalpha]';
 
% Sideslip
C_Xbeta = 0;
C_Ybeta = 0;
C_Zbeta = 0;
C_lbeta = 0;
C_mbeta = 0;
C_nbeta = 0;
C_beta = [C_Xbeta,C_Ybeta,C_Zbeta,C_lbeta,C_mbeta,C_nbeta]';

%Roll Rate
C_Xp = 0;
C_Yp = 0;
C_Zp = 0;
C_mp = 0;
C_lp = -3/32;%*abs(p);
C_np = 0;
C_p = [C_Xp,C_Yp,C_Zp,C_lp,C_mp,C_np]';


% Pitch Rate
C_Xq = 0;
C_Yq = 0;
C_Zq = 0;
C_lq = 0;
C_mq = 0;
C_nq = 0;
C_q = [C_Xq,C_Yq,C_Zq,C_lq,C_mq,C_nq]';

% Yaw Rate
C_Xr = 0;
C_Yr = 0;
C_Zr = 0;
C_lr = 0;
C_mr = 0;
C_nr = 0;
C_r = [C_Xr,C_Yr,C_Zr,C_lr,C_mr,C_nr]';

% % Roll Acceleration
% C_Xpdot = 0;
% C_Ypdot = 0;
% C_Zpdot = 0;
% C_mpdot = 0;
% C_lpdot = -1/32;
% C_npdot = 0;
% C_pdot = [C_Xpdot,C_Ypdot,C_Zpdot,C_lpdot,C_mpdot,C_npdot]';
% 
% % Pitch Acceleration
% C_Xqdot = 0;
% C_Yqdot = 0;
% C_Zqdot = 0;
% C_mqdot = 0;
% C_lqdot = 0;
% C_nqdot = 0;
% C_qdot = [C_Xqdot,C_Yqdot,C_Zqdot,C_lqdot,C_mqdot,C_nqdot]';
% 
% % Yaw Acceleration
% C_Xrdot = 0;
% C_Yrdot = 0;
% C_Zrdot = 0;
% C_mrdot = 0;
% C_lrdot = 0;
% C_nrdot = 0;
% C_rdot = [C_Xrdot,C_Yrdot,C_Zrdot,C_lrdot,C_mrdot,C_nrdot]';

% Combined
A = [C_delta,C_alpha,C_beta,C_p,C_q,C_r];
% A = [C_delta,C_alpha,C_beta,C_p,C_q,C_r,C_pdot,C_qdot,C_rdot];
C = A*x;

if alpha == 0
    C = C+C_alpha;
end

F = C(1:3);
M = C(4:end);

end

== matlab function Potoo_Dyn_Model_v3px4_Flap_compact/Controller/Attitude Controller/MATLAB Function1 ==
  data: body_unit input; body_unit output
function body_unit = limitTilt(body_unit)

orientation_product = dot(body_unit,[0 0 1]');
orientation_angel = acosd(orientation_product);
orientation_angel = min([orientation_angel,45]);

rejection = body_unit-orientation_product*[0 0 1]';
rejection_norm_squared = dot(rejection,rejection);
if rejection_norm_squared == 0
    rejection(1) = 1;
end

body_unit = cosd(orientation_angel)*[0 0 1]'+sind(orientation_angel)*rejection;

== matlab function Potoo_Dyn_Model_v3px4_Flap_compact/Controller/MATLAB Function1 ==
  settings: updateMethod=DISCRETE
  data: theta input; theta output; mission input; t input
function theta = pitch_att_singlet(theta,mission,t)

persistent t_flag state
if isempty(t_flag)
    t_flag = t;
    state = 0;
end

t_on = 0.4703;
theta_target = 25*pi/180;

if mission == 3
    switch state
        case 0
            theta = 0;
            if t >= t_flag+1.6793
                state = 1;
                t_flag = t;
            end
        case 1
            theta = theta_target*sin(2*pi/(2*t_on)*(t-t_flag));
            if t >= t_flag+t_on
                state = 3;
                t_flag = t;
            end
        case 3
            theta = 0;
    end
end
